simulink model "adv_lag_igual_simulink"  (R2016a)
settings: Solver=VariableStepAuto  StartTime=0.0  StopTime=10.0  RelTol=1e-3
values from neighbouring files (symbols this model uses):
  Kc = Kp_desejado/Kp_antigo    (= 99)    [adv_lag_igual.m]    (also in advance_and_lagging_compensator.m = (1)/abs(((s1+zero_adv)/(s1+polo_adv))*planta); advance_compensator.m = (1)/abs(((s1+zero_cont1)/(s1+polo_cont1))*planta); lagging_compensator.m = (1)/abs(((s1+zero_lag)/(s1+polo_lag))*planta))
  polo_adv = 39.8730    (= 39.873)    [adv_lag_igual.m]    (also in advance_and_lagging_compensator.m = sigma + wd*tand(-deficiencia_angular))
  polo_lag = 1/(beta*T2)    (= 0.0702229578913)    [adv_lag_igual.m]    (also in advance_and_lagging_compensator.m = 1/(beta*T2); lagging_compensator.m = 1/(beta*T))
  zero_adv = 4    [adv_lag_igual.m]    (also in advance_and_lagging_compensator.m = abs(max(polos_planta)))
  zero_lag = 0.7    [adv_lag_igual.m]    (also in advance_and_lagging_compensator.m = input('Escolha um Zero para o controlador perto da Origem-> ; lagging_compensator.m = input('Escolha um Zero para o controlador PERTO DE ZERO-> '))
settings Model: Creator=jessa  LastModifiedBy=jessa

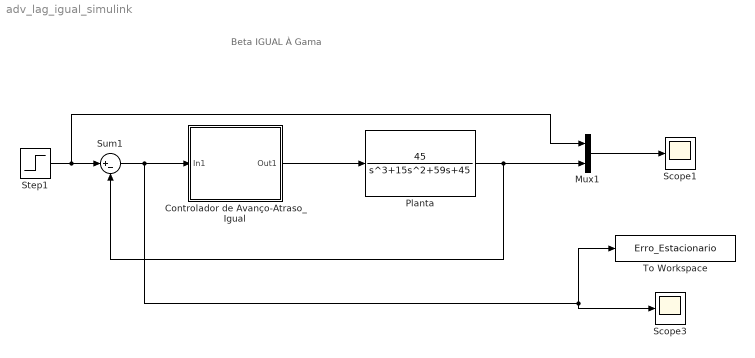
== system adv_lag_igual_simulink ==
  note: Beta IGUAL À Gama
  Controlador de Avanço-Atraso_Igual : Subsystem
  Mux1 : Mux  Inputs=2
  Planta : TransferFcn  Numerator=[45]  Denominator=[1 15 59 45]
  Scope1 : Scope
  Scope3 : Scope
  Step1 : Step  Time=0  SampleTime=0
  Sum1 : Sum  Inputs=|+-
  To Workspace : ToWorkspace  VariableName=Erro_Estacionario  SampleTime=-1
  wires:
  Mux1/1 -> Scope1/1
  Planta/1 -> Sum1/2, Mux1/2
  Step1/1 -> Sum1/1, Mux1/1
  Controlador de Avanço-Atraso_Igual/1(Out1) -> Planta/1
  Sum1/1 -> To Workspace/1, Scope3/1, Controlador de Avanço-Atraso_Igual/1(In1)

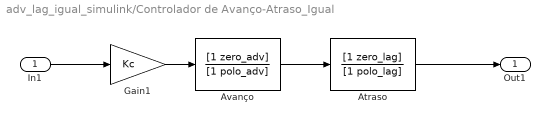
== system adv_lag_igual_simulink/Controlador de Avanço-Atraso_Igual ==
  In1 : Inport
  Atraso : TransferFcn  Numerator=[1 zero_lag]  Denominator=[1 polo_lag]
  Avanço : TransferFcn  Numerator=[1 zero_adv]  Denominator=[1 polo_adv]
  Gain1 : Gain  Gain=Kc
  Out1 : Outport
  wires:
  Atraso/1 -> Out1/1
  In1/1 -> Gain1/1
  Gain1/1 -> Avanço/1
  Avanço/1 -> Atraso/1
